simulink model "ACC_ModeManager_Model"  (R2024b)
settings: Solver=VariableStepAuto  StartTime=0.0  StopTime=10.0  RelTol=1e-3
settings Model: Creator=LENOVO  LastModifiedBy=LENOVO

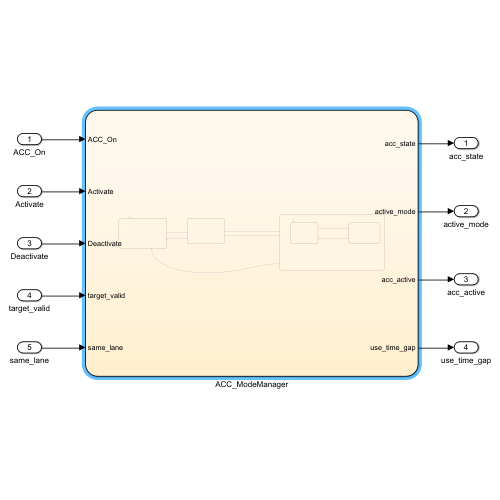
[thumbnail: Simulink's stored preview of the top-level diagram]
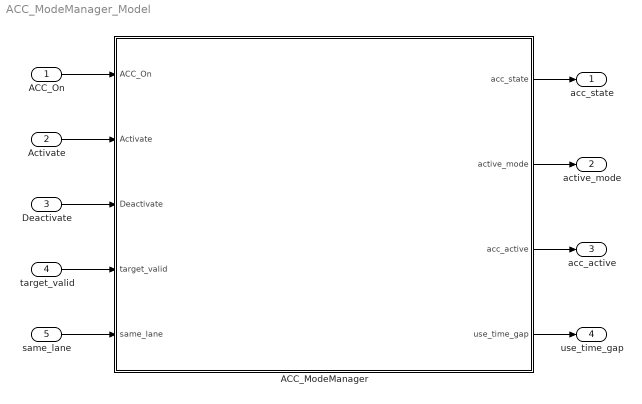
== system ACC_ModeManager_Model ==
  ACC_On : Inport
  Activate : Inport  Port=2
  Deactivate : Inport  Port=3
  target_valid : Inport  Port=4
  same_lane : Inport  Port=5
  ACC_ModeManager : Stateflow chart  TreatAsAtomicUnit=on
  acc_state : Outport
  active_mode : Outport  Port=2
  acc_active : Outport  Port=3
  use_time_gap : Outport  Port=4
  wires:
  Activate/1 -> ACC_ModeManager/2(Activate)
  same_lane/1 -> ACC_ModeManager/5(same_lane)
  ACC_ModeManager/3(acc_active) -> acc_active/1
  target_valid/1 -> ACC_ModeManager/4(target_valid)
  ACC_ModeManager/2(active_mode) -> active_mode/1
  ACC_On/1 -> ACC_ModeManager/1(ACC_On)
  ACC_ModeManager/1(acc_state) -> acc_state/1
  Deactivate/1 -> ACC_ModeManager/3(Deactivate)
  ACC_ModeManager/4(use_time_gap) -> use_time_gap/1

== stateflow chart ACC_ModeManager_Model/ACC_ModeManager ==
  state ACC_Active
    state SpeedControl
      entry:
      mode_changed = true;
      during:
      active_mode  = uint8(1);
      use_time_gap = false;
      mode_changed = false;
      exit:
      ;
    state TimeGapControl
      entry:
      mode_changed = true;
      during:
      active_mode  = uint8(2);
      use_time_gap = true;
      mode_changed = false;
      exit:
      ;
    (default) -> SpeedControl
    SpeedControl -> TimeGapControl : [target_valid && same_lane]
    TimeGapControl -> SpeedControl : [~(target_valid && same_lane)]
  state ACC_Off
    entry:
    mode_changed = true;
    during:
    acc_state    = uint8(0);
    acc_active   = false;
    active_mode  = uint8(0);
    use_time_gap = false;
    mode_changed = false;
    exit:
    ;
  state ACC_Standby
    entry:
    mode_changed = true;
    during:
    acc_state    = uint8(1);
    acc_active   = false;
    active_mode  = uint8(0);
    use_time_gap = false;
    mode_changed = false;
    exit:
    ;
  (default) -> ACC_Off
  ACC_Standby -> ACC_Active [order 2] : [Activate]
  ACC_Off -> ACC_Standby : [ACC_On]
  ACC_Active -> ACC_Standby [order 1] : [Deactivate]
  ACC_Standby -> ACC_Off [order 1] : [~ACC_On]
  ACC_Active -> ACC_Off [order 2] : [~ACC_On]
  data: ACC_On input boolean; Activate input boolean; Deactivate input boolean; target_valid input boolean; same_lane input boolean; acc_state output uint8; active_mode output uint8; acc_active output boolean; use_time_gap output boolean
